simulink model "testinggrounds"  (R2019b)
settings: Solver=VariableStepAuto  StartTime=0.0  StopTime=10.0  RelTol=1e-3
undefined symbols (not defined in the file or in its folder): sdlk
libraries: commrandsrc3 x1, commrflib2 x1, commdigbbndfm2 x1
settings Model: Creator=russe  LastModifiedBy=russe

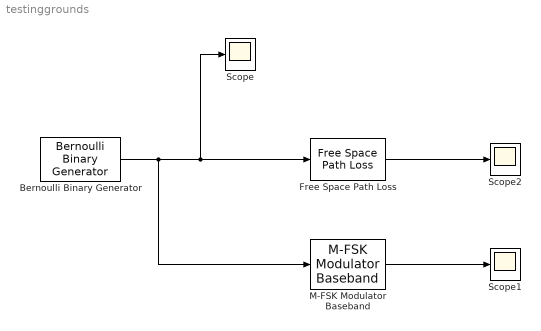
== system testinggrounds ==
  Bernoulli Binary Generator : commrandsrc3/Bernoulli Binary Generator  ProbabilityOfZero=0.5  SeedSource=Auto  Seed=0  SampleTime=sdlk.datarate  SamplesPerFrame=sdlk.bitsperframe  OutputDataType=double  SimulateUsing=Interpreted execution
      settings: SourceProductName=Communications Toolbox
  Free Space Path Loss : commrflib2/Free Space Path Loss  mode=Distance and Frequency  dB=10  d=sdlk.altitude  fc=sdlk.carrierfrequency
      settings: SourceProductName=Communications Toolbox  SourceProductBaseCode=CM
  M-FSK Modulator Baseband : commdigbbndfm2/M-FSK Modulator Baseband  M=4  InType=Integer  Enc=Gray  freqSep=sdlk.deltaf  phaseType=Continuous  numSamp=2  RateOptions=Enforce single-rate processing  outDataType=double
      settings: SourceProductName=Communications Toolbox
  Scope : Scope
  Scope1 : Scope
  Scope2 : Scope
  wires:
  Bernoulli Binary Generator/1 -> M-FSK Modulator Baseband/1, Scope/1, Free Space Path Loss/1
  Free Space Path Loss/1 -> Scope2/1
  M-FSK Modulator Baseband/1 -> Scope1/1
